simulink model "COMPONENT_MDL_Lag_QUAD_and_PEND_with_Ab"  (R2020b)
(part 5 of 12)

(m_pend.*(Ly_pend.^2./1.2e+1+Lz_pend.^2./1.2e+1).*(sin(THE_Psi).*sin(THE_Theta_pend)+cos(THE_Psi).*cos(THE_Theta_pend).*sin(THE_Phi_pend)))./2.0+m_pend.*(Ly_pend.^2./1.2e+1+Lz_pend.^2./1.2e+1).*((sin(THE_Psi).*sin(THE_Theta_pend))./2.0+(cos(THE_Psi).*cos(THE_Theta_pend).*sin(THE_Phi_pend))./2.0)-m_pend.*((Lz_pend.*cos(THE_Phi).*sin(THE_Theta).*(sin(THE_Phi_pend).*sin(THE_Psi_pend)+cos(THE_Phi_pend).*cos(THE_Psi_pend).*sin(THE_Theta_pend)))./2.0-cos(THE_Phi).*cos(THE_Psi).*cos(THE_Theta).*(Tv_Z_pend+(Lz_pend.*cos(THE_Psi_pend).*cos(THE_Theta_pend))./2.0)+(Lz_pend.*cos(THE_Phi).*cos(THE_Theta).*sin(THE_Psi).*(cos(THE_Phi_pend).*sin(THE_Psi_pend)-cos(THE_Psi_pend).*sin(THE_Phi_pend).*sin(THE_Theta_pend)))./2.0).*((Lz_pend.*(cos(THE_Psi).*sin(THE_Phi)-cos(THE_Phi).*sin(THE_Psi).*sin(THE_Theta)).*(cos(THE_Phi_pend).*cos(THE_Psi_pend)+sin(THE_Phi_pend).*sin(THE_Psi_pend).*sin(THE_Theta_pend)))./4.0+(Lz_pend.*cos(THE_Phi).*cos(THE_Theta).*(cos(THE_Psi_pend).*sin(THE_Phi_pend)-cos(THE_Phi_pend).*sin(THE_Psi_pend).*sin(THE_Theta_pend)))./4.0-(Lz_pend.*cos(THE_Theta_pend).*sin(THE_Psi_pend).*(sin(THE_Phi).*sin(THE_Psi)+cos(THE_Phi).*cos(THE_Psi).*sin(THE_Theta)))./4.0)-m_pend.*((Lz_pend.*cos(THE_Phi).*sin(THE_Theta).*(sin(THE_Phi_pend).*sin(THE_Psi_pend)+cos(THE_Phi_pend).*cos(THE_Psi_pend).*sin(THE_Theta_pend)))./4.0-(cos(THE_Phi).*cos(THE_Psi).*cos(THE_Theta).*(Tv_Z_pend+(Lz_pend.*cos(THE_Psi_pend).*cos(THE_Theta_pend))./2.0))./2.0+(Lz_pend.*cos(THE_Phi).*cos(THE_Theta).*sin(THE_Psi).*(cos(THE_Phi_pend).*sin(THE_Psi_pend)-cos(THE_Psi_pend).*sin(THE_Phi_pend).*sin(THE_Theta_pend)))./4.0).*((Lz_pend.*(cos(THE_Psi).*sin(THE_Phi)-cos(THE_Phi).*sin(THE_Psi).*sin(THE_Theta)).*(cos(THE_Phi_pend).*cos(THE_Psi_pend)+sin(THE_Phi_pend).*sin(THE_Psi_pend).*sin(THE_Theta_pend)))./2.0+(Lz_pend.*cos(THE_Phi).*cos(THE_Theta).*(cos(THE_Psi_pend).*sin(THE_Phi_pend)-cos(THE_Phi_pend).*sin(THE_Psi_pend).*sin(THE_Theta_pend)))./2.0-(Lz_pend.*cos(THE_Theta_pend).*sin(THE_Psi_pend).*(sin(THE_Phi).*sin(THE_Psi)+cos(THE_Phi).*cos(THE_Psi).*sin(THE_Theta)))./2.0)-m_pend.*((Lz_pend.*sin(THE_Phi).*sin(THE_Theta).*(sin(THE_Phi_pend).*sin(THE_Psi_pend)+cos(THE_Phi_pend).*cos(THE_Psi_pend).*sin(THE_Theta_pend)))./2.0-cos(THE_Psi).*cos(THE_Theta).*sin(THE_Phi).*(Tv_Z_pend+(Lz_pend.*cos(THE_Psi_pend).*cos(THE_Theta_pend))./2.0)+(Lz_pend.*cos(THE_Theta).*sin(THE_Phi).*sin(THE_Psi).*(cos(THE_Phi_pend).*sin(THE_Psi_pend)-cos(THE_Psi_pend).*sin(THE_Phi_pend).*sin(THE_Theta_pend)))./2.0).*(Lz_pend.*(cos(THE_Phi).*cos(THE_Psi)+sin(THE_Phi).*sin(THE_Psi).*sin(THE_Theta)).*(cos(THE_Phi_pend).*cos(THE_Psi_pend)+sin(THE_Phi_pend).*sin(THE_Psi_pend).*sin(THE_Theta_pend)).*(-1.0./4.0)+(Lz_pend.*cos(THE_Theta_pend).*sin(THE_Psi_pend).*(cos(THE_Phi).*sin(THE_Psi)-cos(THE_Psi).*sin(THE_Phi).*sin(THE_Theta)))./4.0+(Lz_pend.*cos(THE_Theta).*sin(THE_Phi).*(cos(THE_Psi_pend).*sin(THE_Phi_pend)-cos(THE_Phi_pend).*sin(THE_Psi_pend).*sin(THE_Theta_pend)))./4.0)-m_pend.*((Lz_pend.*sin(THE_Phi).*sin(THE_Theta).*(sin(THE_Phi_pend).*sin(THE_Psi_pend)+cos(THE_Phi_pend).*cos(THE_Psi_pend).*sin(THE_Theta_pend)))./4.0-(cos(THE_Psi).*cos(THE_Theta).*sin(THE_Phi).*(Tv_Z_pend+(Lz_pend.*cos(THE_Psi_pend).*cos(THE_Theta_pend))./2.0))./2.0+(Lz_pend.*cos(THE_Theta).*sin(THE_Phi).*sin(THE_Psi).*(cos(THE_Phi_pend).*sin(THE_Psi_pend)-cos(THE_Psi_pend).*sin(THE_Phi_pend).*sin(THE_Theta_pend)))./4.0).*(Lz_pend.*(cos(THE_Phi).*cos(THE_Psi)+sin(THE_Phi).*sin(THE_Psi).*sin(THE_Theta)).*(cos(THE_Phi_pend).*cos(THE_Psi_pend)+sin(THE_Phi_pend).*sin(THE_Psi_pend).*sin(THE_Theta_pend)).*(-1.0./2.0)+(Lz_pend.*cos(THE_Theta_pend).*sin(THE_Psi_pend).*(cos(THE_Phi).*sin(THE_Psi)-cos(THE_Psi).*sin(THE_Phi).*sin(THE_Theta)))./2.0+(Lz_pend.*cos(THE_Theta).*sin(THE_Phi).*(cos(THE_Psi_pend).*sin(THE_Phi_pend)-cos(THE_Phi_pend).*sin(THE_Psi_pend).*sin(THE_Theta_pend)))./2.0)+m_pend.*((Lz_pend.*sin(THE_Theta).*(cos(THE_Psi_pend).*sin(THE_Phi_pend)-cos(THE_Phi_pend).*sin(THE_Psi_pend).*sin(THE_Theta_pend)))./4.0+(Lz_pend.*cos(THE_Theta).*sin(THE_Psi).*(cos(THE_Phi_pend).*cos(THE_Psi_pend)+sin(THE_Phi_pend).*sin(THE_Psi_pend).*sin(THE_Theta_pend)))./4.0+(Lz_pend.*cos(THE_Psi).*cos(THE_Theta).*cos(THE_Theta_pend).*sin(THE_Psi_pend))./4.0).*((Lz_pend.*cos(THE_Theta).*(sin(THE_Phi_pend).*sin(THE_Psi_pend)+cos(THE_Phi_pend).*cos(THE_Psi_pend).*sin(THE_Theta_pend)))./2.0+cos(THE_Psi).*sin(THE_Theta).*(Tv_Z_pend+(Lz_pend.*cos(THE_Psi_pend).*cos(THE_Theta_pend))./2.0)-(Lz_pend.*sin(THE_Psi).*sin(THE_Theta).*(cos(THE_Phi_pend).*sin(THE_Psi_pend)-cos(THE_Psi_pend).*sin(THE_Phi_pend).*sin(THE_Theta_pend)))./2.0)+m_pend.*((Lz_pend.*sin(THE_Theta).*(cos(THE_Psi_pend).*sin(THE_Phi_pend)-cos(THE_Phi_pend).*sin(THE_Psi_pend).*sin(THE_Theta_pend)))./2.0+(Lz_pend.*cos(THE_Theta).*sin(THE_Psi).*(cos(THE_Phi_pend).*cos(THE_Psi_pend)+sin(THE_Phi_pend).*sin(THE_Psi_pend).*sin(THE_Theta_pend)))./2.0+(Lz_pend.*cos(THE_Psi).*cos(THE_Theta).*cos(THE_Theta_pend).*sin(THE_Psi_pend))./2.0).*((Lz_pend.*cos(THE_Theta).*(sin(THE_Phi_pend).*sin(THE_Psi_pend)+cos(THE_Phi_pend).*cos(THE_Psi_pend).*sin(THE_Theta_pend)))./4.0+(cos(THE_Psi).*sin(THE_Theta).*(Tv_Z_pend+(Lz_pend.*cos(THE_Psi_pend).*cos(THE_Theta_pend))./2.0))./2.0-(Lz_pend.*sin(THE_Psi).*sin(THE_Theta).*(cos(THE_Phi_pend).*sin(THE_Psi_pend)-cos(THE_Psi_pend).*sin(THE_Phi_pend).*sin(THE_Theta_pend)))./4.0),m_pend.*((cos(THE_Theta).*sin(THE_Psi).*(Tv_Z_pend+(Lz_pend.*cos(THE_Psi_pend).*cos(THE_Theta_pend))./2.0))./2.0+(Lz_pend.*cos(THE_Psi).*cos(THE_Theta).*(cos(THE_Phi_pend).*sin(THE_Psi_pend)-cos(THE_Psi_pend).*sin(THE_Phi_pend).*sin(THE_Theta_pend)))./4.0).*((Lz_pend.*sin(THE_Theta).*(cos(THE_Psi_pend).*sin(THE_Phi_pend)-cos(THE_Phi_pend).*sin(THE_Psi_pend).*sin(THE_Theta_pend)))./2.0+(Lz_pend.*cos(THE_Theta).*sin(THE_Psi).*(cos(THE_Phi_pend).*cos(THE_Psi_pend)+sin(THE_Phi_pend).*sin(THE_Psi_pend).*sin(THE_Theta_pend)))./2.0+(Lz_pend.*cos(THE_Psi).*cos(THE_Theta).*cos(THE_Theta_pend).*sin(THE_Psi_pend))./2.0)+m_pend.*(cos(THE_Theta).*sin(THE_Psi).*(Tv_Z_pend+(Lz_pend.*cos(THE_Psi_pend).*cos(THE_Theta_pend))./2.0)+(Lz_pend.*cos(THE_Psi).*cos(THE_Theta).*(cos(THE_Phi_pend).*sin(THE_Psi_pend)-cos(THE_Psi_pend).*sin(THE_Phi_pend).*sin(THE_Theta_pend)))./2.0).*((Lz_pend.*sin(THE_Theta).*(cos(THE_Psi_pend).*sin(THE_Phi_pend)-cos(THE_Phi_pend).*sin(THE_Psi_pend).*sin(THE_Theta_pend)))./4.0+(Lz_pend.*cos(THE_Theta).*sin(THE_Psi).*(cos(THE_Phi_pend).*cos(THE_Psi_pend)+sin(THE_Phi_pend).*sin(THE_Psi_pend).*sin(THE_Theta_pend)))./4.0+(Lz_pend.*cos(THE_Psi).*cos(THE_Theta).*cos(THE_Theta_pend).*sin(THE_Psi_pend))./4.0)+m_pend.*(((Tv_Z_pend+(Lz_pend.*cos(THE_Psi_pend).*cos(THE_Theta_pend))./2.0).*(cos(THE_Psi).*sin(THE_Phi)-cos(THE_Phi).*sin(THE_Psi).*sin(THE_Theta)))./2.0-(Lz_pend.*(sin(THE_Phi).*sin(THE_Psi)+cos(THE_Phi).*cos(THE_Psi).*sin(THE_Theta)).*(cos(THE_Phi_pend).*sin(THE_Psi_pend)-cos(THE_Psi_pend).*sin(THE_Phi_pend).*sin(THE_Theta_pend)))./4.0).*((Lz_pend.*(cos(THE_Psi).*sin(THE_Phi)-cos(THE_Phi).*sin(THE_Psi).*sin(THE_Theta)).*(cos(THE_Phi_pend).*cos(THE_Psi_pend)+sin(THE_Phi_pend).*sin(THE_Psi_pend).*sin(THE_Theta_pend)))./2.0+(Lz_pend.*cos(THE_Phi).*cos(THE_Theta).*(cos(THE_Psi_pend).*sin(THE_Phi_pend)-cos(THE_Phi_pend).*sin(THE_Psi_pend).*sin(THE_Theta_pend)))./2.0-(Lz_pend.*cos(THE_Theta_pend).*sin(THE_Psi_pend).*(sin(THE_Phi).*sin(THE_Psi)+cos(THE_Phi).*cos(THE_Psi).*sin(THE_Theta)))./2.0)+m_pend.*((Tv_Z_pend+(Lz_pend.*cos(THE_Psi_pend).*cos(THE_Theta_pend))./2.0).*(cos(THE_Psi).*sin(THE_Phi)-cos(THE_Phi).*sin(THE_Psi).*sin(THE_Theta))-(Lz_pend.*(sin(THE_Phi).*sin(THE_Psi)+cos(THE_Phi).*cos(THE_Psi).*sin(THE_Theta)).*(cos(THE_Phi_pend).*sin(THE_Psi_pend)-cos(THE_Psi_pend).*sin(THE_Phi_pend).*sin(THE_Theta_pend)))./2.0).*((Lz_pend.*(cos(THE_Psi).*sin(THE_Phi)-cos(THE_Phi).*sin(THE_Psi).*sin(THE_Theta)).*(cos(THE_Phi_pend).*cos(THE_Psi_pend)+sin(THE_Phi_pend).*sin(THE_Psi_pend).*sin(THE_Theta_pend)))./4.0+(Lz_pend.*cos(THE_Phi).*cos(THE_Theta).*(cos(THE_Psi_pend).*sin(THE_Phi_pend)-cos(THE_Phi_pend).*sin(THE_Psi_pend).*sin(THE_Theta_pend)))./4.0-(Lz_pend.*cos(THE_Theta_pend).*sin(THE_Psi_pend).*(sin(THE_Phi).*sin(THE_Psi)+cos(THE_Phi).*cos(THE_Psi).*sin(THE_Theta)))./4.0)-m_pend.*(((Tv_Z_pend+(Lz_pend.*cos(THE_Psi_pend).*cos(THE_Theta_pend))./2.0).*(cos(THE_Phi).*cos(THE_Psi)+sin(THE_Phi).*sin(THE_Psi).*sin(THE_Theta)))./2.0-(Lz_pend.*(cos(THE_Phi).*sin(THE_Psi)-cos(THE_Psi).*sin(THE_Phi).*sin(THE_Theta)).*(cos(THE_Phi_pend).*sin(THE_Psi_pend)-cos(THE_Psi_pend).*sin(THE_Phi_pend).*sin(THE_Theta_pend)))./4.0).*(Lz_pend.*(cos(THE_Phi).*cos(THE_Psi)+sin(THE_Phi).*sin(THE_Psi).*sin(THE_Theta)).*(cos(THE_Phi_pend).*cos(THE_Psi_pend)+sin(THE_Phi_pend).*sin(THE_Psi_pend).*sin(THE_Theta_pend)).*(-1.0./2.0)+(Lz_pend.*cos(THE_Theta_pend).*sin(THE_Psi_pend).*(cos(THE_Phi).*sin(THE_Psi)-cos(THE_Psi).*sin(THE_Phi).*sin(THE_Theta)))./2.0+(Lz_pend.*cos(THE_Theta).*sin(THE_Phi).*(cos(THE_Psi_pend).*sin(THE_Phi_pend)-cos(THE_Phi_pend).*sin(THE_Psi_pend).*sin(THE_Theta_pend)))./2.0)-m_pend.*((Tv_Z_pend+(Lz_pend.*cos(THE_Psi_pend).*cos(THE_Theta_pend))./2.0).*(cos(THE_Phi).*cos(THE_Psi)+sin(THE_Phi).*sin(THE_Psi).*sin(THE_Theta))-(Lz_pend.*(cos(THE_Phi).*sin(THE_Psi)-cos(THE_Psi).*sin(THE_Phi).*sin(THE_Theta)).*(cos(THE_Phi_pend).*sin(THE_Psi_pend)-cos(THE_Psi_pend).*sin(THE_Phi_pend).*sin(THE_Theta_pend)))./2.0).*(Lz_pend.*(cos(THE_Phi).*cos(THE_Psi)+sin(THE_Phi).*sin(THE_Psi).*sin(THE_Theta)).*(cos(THE_Phi_pend).*cos(THE_Psi_pend)+sin(THE_Phi_pend).*sin(THE_Psi_pend).*sin(THE_Theta_pend)).*(-1.0./4.0)+(Lz_pend.*cos(THE_Theta_pend).*sin(THE_Psi_pend).*(cos(THE_Phi).*sin(THE_Psi)-cos(THE_Psi).*sin(THE_Phi).*sin(THE_Theta)))./4.0+(Lz_pend.*cos(THE_Theta).*sin(THE_Phi).*(cos(THE_Psi_pend).*sin(THE_Phi_pend)-cos(THE_Phi_pend).*sin(THE_Psi_pend).*sin(THE_Theta_pend)))./4.0)+m_pend.*cos(THE_Phi_pend).*cos(THE_Theta_pend).*(Ly_pend.^2./1.2e+1+Lz_pend.^2./1.2e+1),(m_pend.*((Lz_pend.*(cos(THE_Psi).*sin(THE_Phi)-cos(THE_Phi).*sin(THE_Psi).*sin(THE_Theta)).*(cos(THE_Phi_pend).*cos(THE_Psi_pend)+sin(THE_Phi_pend).*sin(THE_Psi_pend).*sin(THE_Theta_pend)))./2.0+(Lz_pend.*cos(THE_Phi).*cos(THE_Theta).*(cos(THE_Psi_pend).*sin(THE_Phi_pend)-cos(THE_Phi_pend).*sin(THE_Psi_pend).*sin(THE_Theta_pend)))./2.0-(Lz_pend.*cos(THE_Theta_pend).*sin(THE_Psi_pend).*(sin(THE_Phi).*sin(THE_Psi)+cos(THE_Phi).*cos(THE_Psi).*sin(THE_Theta)))./2.0))./2.0+m_pend.*((Lz_pend.*(cos(THE_Psi).*sin(THE_Phi)-cos(THE_Phi).*sin(THE_Psi).*sin(THE_Theta)).*(cos(THE_Phi_pend).*cos(THE_Psi_pend)+sin(THE_Phi_pend).*sin(THE_Psi_pend).*sin(THE_Theta_pend)))./4.0+(Lz_pend.*cos(THE_Phi).*cos(THE_Theta).*(cos(THE_Psi_pend).*sin(THE_Phi_pend)-cos(THE_Phi_pend).*sin(THE_Psi_pend).*sin(THE_Theta_pend)))./4.0-(Lz_pend.*cos(THE_Theta_pend).*sin(THE_Psi_pend).*(sin(THE_Phi).*sin(THE_Psi)+cos(THE_Phi).*cos(THE_Psi).*sin(THE_Theta)))./4.0),(m_pend.*(Lz_pend.*(cos(THE_Phi).*cos(THE_Psi)+sin(THE_Phi).*sin(THE_Psi).*sin(THE_Theta)).*(cos(THE_Phi_pend).*cos(THE_Psi_pend)+sin(THE_Phi_pend).*sin(THE_Psi_pend).*sin(THE_Theta_pend)).*(-1.0./2.0)+(Lz_pend.*cos(THE_Theta_pend).*sin(THE_Psi_pend).*(cos(THE_Phi).*sin(THE_Psi)-cos(THE_Psi).*sin(THE_Phi).*sin(THE_Theta)))./2.0+(Lz_pend.*cos(THE_Theta).*sin(THE_Phi).*(cos(THE_Psi_pend).*sin(THE_Phi_pend)-cos(THE_Phi_pend).*sin(THE_Psi_pend).*sin(THE_Theta_pend)))./2.0))./2.0+m_pend.*(Lz_pend.*(cos(THE_Phi).*cos(THE_Psi)+sin(THE_Phi).*sin(THE_Psi).*sin(THE_Theta)).*(cos(THE_Phi_pend).*cos(THE_Psi_pend)+sin(THE_Phi_pend).*sin(THE_Psi_pend).*sin(THE_Theta_pend)).*(-1.0./4.0)+(Lz_pend.*cos(THE_Theta_pend).*sin(THE_Psi_pend).*(cos(THE_Phi).*sin(THE_Psi)-cos(THE_Psi).*sin(THE_Phi).*sin(THE_Theta)))./4.0+(Lz_pend.*cos(THE_Theta).*sin(THE_Phi).*(cos(THE_Psi_pend).*sin(THE_Phi_pend)-cos(THE_Phi_pend).*sin(THE_Psi_pend).*sin(THE_Theta_pend)))./4.0),m_pend.*((Lz_pend.*sin(THE_Theta).*(cos(THE_Psi_pend).*sin(THE_Phi_pend)-cos(THE_Phi_pend).*sin(THE_Psi_pend).*sin(THE_Theta_pend)))./2.0+(Lz_pend.*cos(THE_Theta).*sin(THE_Psi).*(cos(THE_Phi_pend).*cos(THE_Psi_pend)+sin(THE_Phi_pend).*sin(THE_Psi_pend).*sin(THE_Theta_pend)))./2.0+(Lz_pend.*cos(THE_Psi).*cos(THE_Theta).*cos(THE_Theta_pend).*sin(THE_Psi_pend))./2.0).*(-1.0./2.0)-m_pend.*((Lz_pend.*sin(THE_Theta).*(cos(THE_Psi_pend).*sin(THE_Phi_pend)-cos(THE_Phi_pend).*sin(THE_Psi_pend).*sin(THE_Theta_pend)))./4.0+(Lz_pend.*cos(THE_Theta).*sin(THE_Psi).*(cos(THE_Phi_pend).*cos(THE_Psi_pend)+sin(THE_Phi_pend).*sin(THE_Psi_pend).*sin(THE_Theta_pend)))./4.0+(Lz_pend.*cos(THE_Psi).*cos(THE_Theta).*cos(THE_Theta_pend).*sin(THE_Psi_pend))./4.0),-m_pend.*sin(THE_Theta_pend).*(Ly_pend.^2./1.2e+1+Lz_pend.^2./1.2e+1)-m_pend.*((Lz_pend.*(cos(THE_Psi).*sin(THE_Phi)-cos(THE_Phi).*sin(THE_Psi).*sin(THE_Theta)).*(sin(THE_Phi_pend).*sin(THE_Psi_pend)+cos(THE_Phi_pend).*cos(THE_Psi_pend).*sin(THE_Theta_pend)))./4.0-(Lz_pend.*cos(THE_Phi).*cos(THE_Theta).*(cos(THE_Phi_pend).*sin(THE_Psi_pend)-cos(THE_Psi_pend).*sin(THE_Phi_pend).*sin(THE_Theta_pend)))./4.0).*((Lz_pend.*(cos(THE_Psi).*sin(THE_Phi)-cos(THE_Phi).*sin(THE_Psi).*sin(THE_Theta)).*(cos(THE_Phi_pend).*cos(THE_Psi_pend)+sin(THE_Phi_pend).*sin(THE_Psi_pend).*sin(THE_Theta_pend)))./2.0+(Lz_pend.*cos(THE_Phi).*cos(THE_Theta).*(cos(THE_Psi_pend).*sin(THE_Phi_pend)-cos(THE_Phi_pend).*sin(THE_Psi_pend).*sin(THE_Theta_pend)))./2.0-(Lz_pend.*cos(THE_Theta_pend).*sin(THE_Psi_pend).*(sin(THE_Phi).*sin(THE_Psi)+cos(THE_Phi).*cos(THE_Psi).*sin(THE_Theta)))./2.0)-m_pend.*((Lz_pend.*(cos(THE_Psi).*sin(THE_Phi)-cos(THE_Phi).*sin(THE_Psi).*sin(THE_Theta)).*(sin(THE_Phi_pend).*sin(THE_Psi_pend)+cos(THE_Phi_pend).*cos(THE_Psi_pend).*sin(THE_Theta_pend)))./2.0-(Lz_pend.*cos(THE_Phi).*cos(THE_Theta).*(cos(THE_Phi_pend).*sin(THE_Psi_pend)-cos(THE_Psi_pend).*sin(THE_Phi_pend).*sin(THE_Theta_pend)))./2.0).*((Lz_pend.*(cos(THE_Psi).*sin(THE_Phi)-cos(THE_Phi).*sin(THE_Psi).*sin(THE_Theta)).*(cos(THE_Phi_pend).*cos(THE_Psi_pend)+sin(THE_Phi_pend).*sin(THE_Psi_pend).*sin(THE_Theta_pend)))./4.0+(Lz_pend.*cos(THE_Phi).*cos(THE_Theta).*(cos(THE_Psi_pend).*sin(THE_Phi_pend)-cos(THE_Phi_pend).*sin(THE_Psi_pend).*sin(THE_Theta_pend)))./4.0-(Lz_pend.*cos(THE_Theta_pend).*sin(THE_Psi_pend).*(sin(THE_Phi).*sin(THE_Psi)+cos(THE_Phi).*cos(THE_Psi).*sin(THE_Theta)))./4.0)+m_pend.*((Lz_pend.*(cos(THE_Phi).*cos(THE_Psi)+sin(THE_Phi).*sin(THE_Psi).*sin(THE_Theta)).*(sin(THE_Phi_pend).*sin(THE_Psi_pend)+cos(THE_Phi_pend).*cos(THE_Psi_pend).*sin(THE_Theta_pend)))./4.0+(Lz_pend.*cos(THE_Theta).*sin(THE_Phi).*(cos(THE_Phi_pend).*sin(THE_Psi_pend)-cos(THE_Psi_pend).*sin(THE_Phi_pend).*sin(THE_Theta_pend)))./4.0).*(Lz_pend.*(cos(THE_Phi).*cos(THE_Psi)+sin(THE_Phi).*sin(THE_Psi).*sin(THE_Theta)).*(cos(THE_Phi_pend).*cos(THE_Psi_pend)+sin(THE_Phi_pend).*sin(THE_Psi_pend).*sin(THE_Theta_pend)).*(-1.0./2.0)+(Lz_pend.*cos(THE_Theta_pend).*sin(THE_Psi_pend).*(cos(THE_Phi).*sin(THE_Psi)-cos(THE_Psi).*sin(THE_Phi).*sin(THE_Theta)))./2.0+(Lz_pend.*cos(THE_Theta).*sin(THE_Phi).*(cos(THE_Psi_pend).*sin(THE_Phi_pend)-cos(THE_Phi_pend).*sin(THE_Psi_pend).*sin(THE_Theta_pend)))./2.0)+m_pend.*((Lz_pend.*(cos(THE_Phi).*cos(THE_Psi)+sin(THE_Phi).*sin(THE_Psi).*sin(THE_Theta)).*(sin(THE_Phi_pend).*sin(THE_Psi_pend)+cos(THE_Phi_pend).*cos(THE_Psi_pend).*sin(THE_Theta_pend)))./2.0+(Lz_pend.*cos(THE_Theta).*sin(THE_Phi).*(cos(THE_Phi_pend).*sin(THE_Psi_pend)-cos(THE_Psi_pend).*sin(THE_Phi_pend).*sin(THE_Theta_pend)))./2.0).*(Lz_pend.*(cos(THE_Phi).*cos(THE_Psi)+sin(THE_Phi).*sin(THE_Psi).*sin(THE_Theta)).*(cos(THE_Phi_pend).*cos(THE_Psi_pend)+sin(THE_Phi_pend).*sin(THE_Psi_pend).*sin(THE_Theta_pend)).*(-1.0./4.0)+(Lz_pend.*cos(THE_Theta_pend).*sin(THE_Psi_pend).*(cos(THE_Phi).*sin(THE_Psi)-cos(THE_Psi).*sin(THE_Phi).*sin(THE_Theta)))./4.0+(Lz_pend.*cos(THE_Theta).*sin(THE_Phi).*(cos(THE_Psi_pend).*sin(THE_Phi_pend)-cos(THE_Phi_pend).*sin(THE_Psi_pend).*sin(THE_Theta_pend)))./4.0)+m_pend.*((Lz_pend.*sin(THE_Theta).*(cos(THE_Phi_pend).*sin(THE_Psi_pend)-cos(THE_Psi_pend).*sin(THE_Phi_pend).*sin(THE_Theta_pend)))./4.0-(Lz_pend.*cos(THE_Theta).*sin(THE_Psi).*(sin(THE_Phi_pend).*sin(THE_Psi_pend)+cos(THE_Phi_pend).*cos(THE_Psi_pend).*sin(THE_Theta_pend)))./4.0).*((Lz_pend.*sin(THE_Theta).*(cos(THE_Psi_pend).*sin(THE_Phi_pend)-cos(THE_Phi_pend).*sin(THE_Psi_pend).*sin(THE_Theta_pend)))./2.0+(Lz_pend.*cos(THE_Theta).*sin(THE_Psi).*(cos(THE_Phi_pend).*cos(THE_Psi_pend)+sin(THE_Phi_pend).*sin(THE_Psi_pend).*sin(THE_Theta_pend)))./2.0+(Lz_pend.*cos(THE_Psi).*cos(THE_Theta).*cos(THE_Theta_pend).*sin(THE_Psi_pend))./2.0)+m_pend.*((Lz_pend.*sin(THE_Theta).*(cos(THE_Phi_pend).*sin(THE_Psi_pend)-cos(THE_Psi_pend).*sin(THE_Phi_pend).*sin(THE_Theta_pend)))./2.0-(Lz_pend.*cos(THE_Theta).*sin(THE_Psi).*(sin(THE_Phi_pend).*sin(THE_Psi_pend)+cos(THE_Phi_pend).*cos(THE_Psi_pend).*sin(THE_Theta_pend)))./2.0).*((Lz_pend.*sin(THE_Theta).*(cos(THE_Psi_pend).*sin(THE_Phi_pend)-cos(THE_Phi_pend).*sin(THE_Psi_pend).*sin(THE_Theta_pend)))./4.0+(Lz_pend.*cos(THE_Theta).*sin(THE_Psi).*(cos(THE_Phi_pend).*cos(THE_Psi_pend)+sin(THE_Phi_pend).*sin(THE_Psi_pend).*sin(THE_Theta_pend)))./4.0+(Lz_pend.*cos(THE_Psi).*cos(THE_Theta).*cos(THE_Theta_pend).*sin(THE_Psi_pend))./4.0),m_pend.*((Lz_pend.*sin(THE_Theta).*(cos(THE_Psi_pend).*sin(THE_Phi_pend)-cos(THE_Phi_pend).*sin(THE_Psi_pend).*sin(THE_Theta_pend)))./2.0+(Lz_pend.*cos(THE_Theta).*sin(THE_Psi).*(cos(THE_Phi_pend).*cos(THE_Psi_pend)+sin(THE_Phi_pend).*sin(THE_Psi_pend).*sin(THE_Theta_pend)))./2.0+(Lz_pend.*cos(THE_Psi).*cos(THE_Theta).*cos(THE_Theta_pend).*sin(THE_Psi_pend))./2.0).*((Lz_pend.*cos(THE_Psi).*cos(THE_Theta).*cos(THE_Psi_pend).*sin(THE_Theta_pend))./4.0+(Lz_pend.*cos(THE_Phi_pend).*cos(THE_Psi_pend).*cos(THE_Theta_pend).*sin(THE_Theta))./4.0-(Lz_pend.*cos(THE_Theta).*cos(THE_Psi_pend).*cos(THE_Theta_pend).*sin(THE_Psi).*sin(THE_Phi_pend))./4.0)+m_pend.*((Lz_pend.*sin(THE_Theta).*(cos(THE_Psi_pend).*sin(THE_Phi_pend)-cos(THE_Phi_pend).*sin(THE_Psi_pend).*sin(THE_Theta_pend)))./4.0+(Lz_pend.*cos(THE_Theta).*sin(THE_Psi).*(cos(THE_Phi_pend).*cos(THE_Psi_pend)+sin(THE_Phi_pend).*sin(THE_Psi_pend).*sin(THE_Theta_pend)))./4.0+(Lz_pend.*cos(THE_Psi).*cos(THE_Theta).*cos(THE_Theta_pend).*sin(THE_Psi_pend))./4.0).*((Lz_pend.*cos(THE_Psi).*cos(THE_Theta).*cos(THE_Psi_pend).*sin(THE_Theta_pend))./2.0+(Lz_pend.*cos(THE_Phi_pend).*cos(THE_Psi_pend).*cos(THE_Theta_pend).*sin(THE_Theta))./2.0-(Lz_pend.*cos(THE_Theta).*cos(THE_Psi_pend).*cos(THE_Theta_pend).*sin(THE_Psi).*sin(THE_Phi_pend))./2.0)-m_pend.*((Lz_pend.*cos(THE_Psi_pend).*sin(THE_Theta_pend).*(sin(THE_Phi).*sin(THE_Psi)+cos(THE_Phi).*cos(THE_Psi).*sin(THE_Theta)))./2.0+(Lz_pend.*cos(THE_Psi_pend).*cos(THE_Theta_pend).*sin(THE_Phi_pend).*(cos(THE_Psi).*sin(THE_Phi)-cos(THE_Phi).*sin(THE_Psi).*sin(THE_Theta)))./2.0-(Lz_pend.*cos(THE_Phi).*cos(THE_Theta).*cos(THE_Phi_pend).*cos(THE_Psi_pend).*cos(THE_Theta_pend))./2.0).*((Lz_pend.*(cos(THE_Psi).*sin(THE_Phi)-cos(THE_Phi).*sin(THE_Psi).*sin(THE_Theta)).*(cos(THE_Phi_pend).*cos(THE_Psi_pend)+sin(THE_Phi_pend).*sin(THE_Psi_pend).*sin(THE_Theta_pend)))./4.0+(Lz_pend.*cos(THE_Phi).*cos(THE_Theta).*(cos(THE_Psi_pend).*sin(THE_Phi_pend)-cos(THE_Phi_pend).*sin(THE_Psi_pend).*sin(THE_Theta_pend)))./4.0-(Lz_pend.*cos(THE_Theta_pend).*sin(THE_Psi_pend).*(sin(THE_Phi).*sin(THE_Psi)+cos(THE_Phi).*cos(THE_Psi).*sin(THE_Theta)))./4.0)-m_pend.*((Lz_pend.*cos(THE_Psi_pend).*sin(THE_Theta_pend).*(sin(THE_Phi).*sin(THE_Psi)+cos(THE_Phi).*cos(THE_Psi).*sin(THE_Theta)))./4.0+(Lz_pend.*cos(THE_Psi_pend).*cos(THE_Theta_pend).*sin(THE_Phi_pend).*(cos(THE_Psi).*sin(THE_Phi)-cos(THE_Phi).*sin(THE_Psi).*sin(THE_Theta)))./4.0-(Lz_pend.*cos(THE_Phi).*cos(THE_Theta).*cos(THE_Phi_pend).*cos(THE_Psi_pend).*cos(THE_Theta_pend))./4.0).*((Lz_pend.*(cos(THE_Psi).*sin(THE_Phi)-cos(THE_Phi).*sin(THE_Psi).*sin(THE_Theta)).*(cos(THE_Phi_pend).*cos(THE_Psi_pend)+sin(THE_Phi_pend).*sin(THE_Psi_pend).*sin(THE_Theta_pend)))./2.0+(Lz_pend.*cos(THE_Phi).*cos(THE_Theta).*(cos(THE_Psi_pend).*sin(THE_Phi_pend)-cos(THE_Phi_pend).*sin(THE_Psi_pend).*sin(THE_Theta_pend)))./2.0-(Lz_pend.*cos(THE_Theta_pend).*sin(THE_Psi_pend).*(sin(THE_Phi).*sin(THE_Psi)+cos(THE_Phi).*cos(THE_Psi).*sin(THE_Theta)))./2.0)+m_pend.*((Lz_pend.*cos(THE_Psi_pend).*sin(THE_Theta_pend).*(cos(THE_Phi).*sin(THE_Psi)-cos(THE_Psi).*sin(THE_Phi).*sin(THE_Theta)))./2.0+(Lz_pend.*cos(THE_Psi_pend).*cos(THE_Theta_pend).*sin(THE_Phi_pend).*(cos(THE_Phi).*cos(THE_Psi)+sin(THE_Phi).*sin(THE_Psi).*sin(THE_Theta)))./2.0+(Lz_pend.*cos(THE_Theta).*cos(THE_Phi_pend).*cos(THE_Psi_pend).*cos(THE_Theta_pend).*sin(THE_Phi))./2.0).*(Lz_pend.*(cos(THE_Phi).*cos(THE_Psi)+sin(THE_Phi).*sin(THE_Psi).*sin(THE_Theta)).*(cos(THE_Phi_pend).*cos(THE_Psi_pend)+sin(THE_Phi_pend).*sin(THE_Psi_pend).*sin(THE_Theta_pend)).*(-1.0./4.0)+(Lz_pend.*cos(THE_Theta_pend).*sin(THE_Psi_pend).*(cos(THE_Phi).*sin(THE_Psi)-cos(THE_Psi).*sin(THE_Phi).*sin(THE_Theta)))./4.0+(Lz_pend.*cos(THE_Theta).*sin(THE_Phi).*(cos(THE_Psi_pend).*sin(THE_Phi_pend)-cos(THE_Phi_pend).*sin(THE_Psi_pend).*sin(THE_Theta_pend)))./4.0)+m_pend.*((Lz_pend.*cos(THE_Psi_pend).*sin(THE_Theta_pend).*(cos(THE_Phi).*sin(THE_Psi)-cos(THE_Psi).*sin(THE_Phi).*sin(THE_Theta)))./4.0+(Lz_pend.*cos(THE_Psi_pend).*cos(THE_Theta_pend).*sin(THE_Phi_pend).*(cos(THE_Phi).*cos(THE_Psi)+sin(THE_Phi).*sin(THE_Psi).*sin(THE_Theta)))./4.0+(Lz_pend.*cos(THE_Theta).*cos(THE_Phi_pend).*cos(THE_Psi_pend).*cos(THE_Theta_pend).*sin(THE_Phi))./4.0).*(Lz_pend.*(cos(THE_Phi).*cos(THE_Psi)+sin(THE_Phi).*sin(THE_Psi).*sin(THE_Theta)).*(cos(THE_Phi_pend).*cos(THE_Psi_pend)+sin(THE_Phi_pend).*sin(THE_Psi_pend).*sin(THE_Theta_pend)).*(-1.0./2.0)+(Lz_pend.*cos(THE_Theta_pend).*sin(THE_Psi_pend).*(cos(THE_Phi).*sin(THE_Psi)-cos(THE_Psi).*sin(THE_Phi).*sin(THE_Theta)))./2.0+(Lz_pend.*cos(THE_Theta).*sin(THE_Phi).*(cos(THE_Psi_pend).*sin(THE_Phi_pend)-cos(THE_Phi_pend).*sin(THE_Psi_pend).*sin(THE_Theta_pend)))./2.0),m_pend.*(Ly_pend.^2./1.2e+1+Lz_pend.^2./1.2e+1)+m_pend.*((Lz_pend.*sin(THE_Theta).*(cos(THE_Psi_pend).*sin(THE_Phi_pend)-cos(THE_Phi_pend).*sin(THE_Psi_pend).*sin(THE_Theta_pend)))./2.0+(Lz_pend.*cos(THE_Theta).*sin(THE_Psi).*(cos(THE_Phi_pend).*cos(THE_Psi_pend)+sin(THE_Phi_pend).*sin(THE_Psi_pend).*sin(THE_Theta_pend)))./2.0+(Lz_pend.*cos(THE_Psi).*cos(THE_Theta).*cos(THE_Theta_pend).*sin(THE_Psi_pend))./2.0).*((Lz_pend.*sin(THE_Theta).*(cos(THE_Psi_pend).*sin(THE_Phi_pend)-cos(THE_Phi_pend).*sin(THE_Psi_pend).*sin(THE_Theta_pend)))./4.0+(Lz_pend.*cos(THE_Theta).*sin(THE_Psi).*(cos(THE_Phi_pend).*cos(THE_Psi_pend)+sin(THE_Phi_pend).*sin(THE_Psi_pend).*sin(THE_Theta_pend)))./4.0+(Lz_pend.*cos(THE_Psi).*cos(THE_Theta).*cos(THE_Theta_pend).*sin(THE_Psi_pend))./4.0).*2.0+m_pend.*((Lz_pend.*(cos(THE_Psi).*sin(THE_Phi)-cos(THE_Phi).*sin(THE_Psi).*sin(THE_Theta)).*(cos(THE_Phi_pend).*cos(THE_Psi_pend)+sin(THE_Phi_pend).*sin(THE_Psi_pend).*sin(THE_Theta_pend)))./2.0+(Lz_pend.*cos(THE_Phi).*cos(THE_Theta).*(cos(THE_Psi_pend).*sin(THE_Phi_pend)-cos(THE_Phi_pend).*sin(THE_Psi_pend).*sin(THE_Theta_pend)))./2.0-(Lz_pend.*cos(THE_Theta_pend).*sin(THE_Psi_pend).*(sin(THE_Phi).*sin(THE_Psi)+cos(THE_Phi).*cos(THE_Psi).*sin(THE_Theta)))./2.0).*((Lz_pend.*(cos(THE_Psi).*sin(THE_Phi)-cos(THE_Phi).*sin(THE_Psi).*sin(THE_Theta)).*(cos(THE_Phi_pend).*cos(THE_Psi_pend)+sin(THE_Phi_pend).*sin(THE_Psi_pend).*sin(THE_Theta_pend)))./4.0+(Lz_pend.*cos(THE_Phi).*cos(THE_Theta).*(cos(THE_Psi_pend).*sin(THE_Phi_pend)-cos(THE_Phi_pend).*sin(THE_Psi_pend).*sin(THE_Theta_pend)))./4.0-(Lz_pend.*cos(THE_Theta_pend).*sin(THE_Psi_pend).*(sin(THE_Phi).*sin(THE_Psi)+cos(THE_Phi).*cos(THE_Psi).*sin(THE_Theta)))./4.0).*2.0+m_pend.*(Lz_pend.*(cos(THE_Phi).*cos(THE_Psi)+sin(THE_Phi).*sin(THE_Psi).*sin(THE_Theta)).*(cos(THE_Phi_pend).*cos(THE_Psi_pend)+sin(THE_Phi_pend).*sin(THE_Psi_pend).*sin(THE_Theta_pend)).*(-1.0./2.0)+(Lz_pend.*cos(THE_Theta_pend).*sin(THE_Psi_pend).*(cos(THE_Phi).*sin(THE_Psi)-cos(THE_Psi).*sin(THE_Phi).*sin(THE_Theta)))./2.0+(Lz_pend.*cos(THE_Theta).*sin(THE_Phi).*(cos(THE_Psi_pend).*sin(THE_Phi_pend)-cos(THE_Phi_pend).*sin(THE_Psi_pend).*sin(THE_Theta_pend)))./2.0).*(Lz_pend.*(cos(THE_Phi).*cos(THE_Psi)+sin(THE_Phi).*sin(THE_Psi).*sin(THE_Theta)).*(cos(THE_Phi_pend).*cos(THE_Psi_pend)+sin(THE_Phi_pend).*sin(THE_Psi_pend).*sin(THE_Theta_pend)).*(-1.0./4.0)+(Lz_pend.*cos(THE_Theta_pend).*sin(THE_Psi_pend).*(cos(THE_Phi).*sin(THE_Psi)-cos(THE_Psi).*sin(THE_Phi).*sin(THE_Theta)))./4.0+(Lz_pend.*cos(THE_Theta).*sin(THE_Phi).*(cos(THE_Psi_pend).*sin(THE_Phi_pend)-cos(THE_Phi_pend).*sin(THE_Psi_pend).*sin(THE_Theta_pend)))./4.0).*2.0],[9,9]);
if nargout > 1
